simulink model "H_inf_simulink"  (R2025b)
settings: Solver=VariableStepAuto  StartTime=0.0  StopTime=100  RelTol=1e-3
values from neighbouring files (symbols this model uses):
  A = [ 0, 1, 0, 0 ... (first row only)    [Controller_LQR.m]    (also in H_inf_controller.m = zeros(4,4); Hinf.m = zeros(4,4); Hinf_tuner.m = zeros(4,4); LQG_controller.m = zeros(4,4))
  B = [0 ... (first row only)    [Controller_LQR.m]    (also in H_inf_controller.m = (dx_p - dx_m) / (2*h); Hinf.m = (dx_p - dx_m) / (2*h); Hinf_tuner.m = (dx_p - dx_m)/(2*h); LQG_controller.m = (dx_p - dx_m) / (2*h))
  C = [1 0 0 0]    [Controller_LQR.m]    (also in H_inf_controller.m; Hinf.m; Hinf_tuner.m; LQG_controller.m)
  D = 0    [Controller_LQR.m]    (also in H_inf_controller.m; Hinf.m; Hinf_tuner.m; LQG_controller.m)
libraries: cstblocks x5, simulink x1
settings Model: Creator=Administrator  LastModifiedBy=Administrator

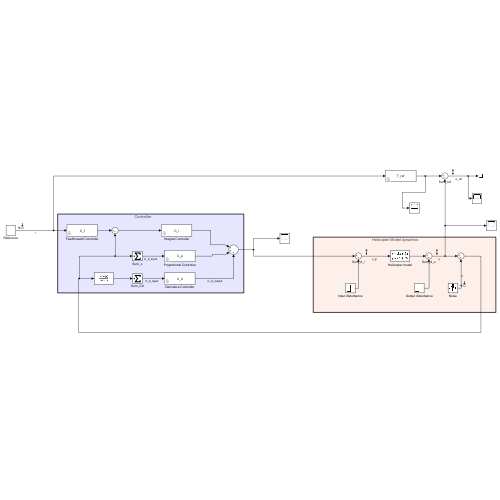
[thumbnail: Simulink's stored preview of the top-level diagram]
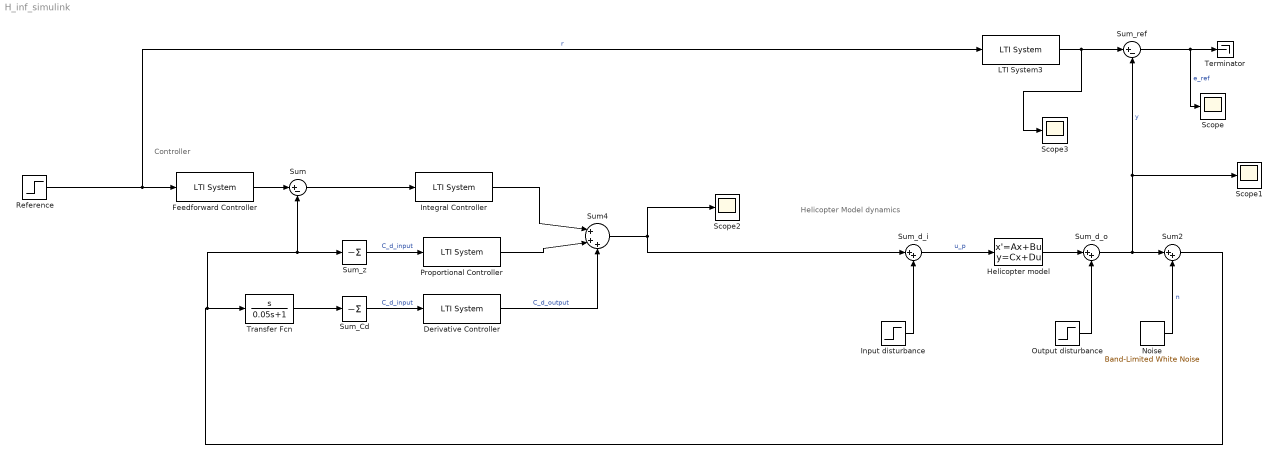
== system H_inf_simulink ==
  note: Controller
  note: Helicopter Model dynamics
  Derivative Controller : cstblocks/LTI System  sys=C_d  IC=[]  PadeOrder=0
  Feedforward Controller : cstblocks/LTI System  sys=C_f  IC=[]  PadeOrder=0
  Helicopter model : StateSpace  A=A  B=B  C=C  D=D  InitialCondition=0
  Input disturbance : Step  After=0  SampleTime=0
  Integral Controller : cstblocks/LTI System  sys=C_i  IC=[]  PadeOrder=0
  LTI System3 : cstblocks/LTI System  sys=T_ref  IC=[]  PadeOrder=0
  Noise : simulink/Sources/Band-Limited White Noise  Cov=[0]  Ts=0.1  seed=[23341]
  Output disturbance : Step  SampleTime=0
  Proportional Controller : cstblocks/LTI System  sys=C_p  IC=[]  PadeOrder=0
  Reference : Step  SampleTime=0
  Scope{,1..3} (4 alike) : Scope
      Scope settings: ActiveDisplayYMinimum=-6.2252239377243965  ActiveDisplayYMaximum=3.5969953594481749
      Scope1 settings: ActiveDisplayYMinimum=-5.95762578986392  ActiveDisplayYMaximum=5.0990816046001921
      Scope2 settings: ActiveDisplayYMinimum=1.0445505252113905  ActiveDisplayYMaximum=2.3982292492687667  DataLoggingVariableName=ScopeData2
      Scope3 settings: ActiveDisplayYMinimum=-1  ActiveDisplayYMaximum=1  DataLoggingVariableName=ScopeData3
  Sum : Sum  Inputs=|+-
  Sum2 : Sum  Inputs=|++
  Sum4 : Sum  Inputs=|+++
  Sum_Cd : Sum  Inputs=-
  Sum_d_i : Sum  Inputs=|++
  Sum_d_o : Sum  Inputs=|++
  Sum_ref : Sum  Inputs=|+-
  Sum_z : Sum  Inputs=-
  Terminator : Terminator
  Transfer Fcn : TransferFcn  Numerator=[1 0]  Denominator=[0.05 1]
  wires:
  Sum_d_i/1 -> Helicopter model/1  "u_p"
  Input disturbance/1 -> Sum_d_i/2
  Helicopter model/1 -> Sum_d_o/1
  Output disturbance/1 -> Sum_d_o/2
  Sum_d_o/1 -> Sum2/1, Sum_ref/2, Scope1/1  "y"
  Noise/1 -> Sum2/2  "n"
  Sum2/1 -> Sum_z/1, Sum/2, Transfer Fcn/1
  Transfer Fcn/1 -> Sum_Cd/1
  Sum_Cd/1 -> Derivative Controller/1  "C_d_input"
  Reference/1 -> Feedforward Controller/1, LTI System3/1  "r"
  Derivative Controller/1 -> Sum4/3  "C_d_output"
  LTI System3/1 -> Scope3/1, Sum_ref/1
  Sum_ref/1 -> Scope/1, Terminator/1  "e_ref"
  Sum4/1 -> Sum_d_i/1, Scope2/1
  Feedforward Controller/1 -> Sum/1
  Sum_z/1 -> Proportional Controller/1  "C_d_input"
  Sum/1 -> Integral Controller/1
  Proportional Controller/1 -> Sum4/2
  Integral Controller/1 -> Sum4/1
